simulink model "MaliLib"  (R2023b)
settings: Solver=FixedStepAuto  StartTime=0.0  StopTime=inf  RelTol=1e-3  EnableMultiTasking=on
settings Model: ExtModeTrigDuration=10  Creator=memoj  LastModifiedBy=memoj
settings OptimizationCC: EnhancedBackFolding=on  PassReuseOutputArgsAs=Individual arguments  ZeroExternalMemoryAtStartup=off  ZeroInternalMemoryAtStartup=off  MaxStackSize=64  OptimizeBlockOrder=speed  DifferentSizesBufferReuse=on  OptimizationCustomize=off  EfficientTunableParamExpr=on
settings DebuggingCC: ParameterTunabilityLossMsg=error
settings HardwareCC: ProdBitPerPointer=32  ProdBitPerSizeT=32  ProdBitPerPtrDiffT=32  ProdLargestAtomicInteger=Long  ProdLargestAtomicFloat=Double  ProdWordSize=32  ProdLongLongMode=on  ProdHWDeviceType=ARM Compatible->ARM Cortex
settings SFSimCC: MATLABDynamicMemAlloc=off
settings RTWCC: Description=Embedded Coder  SystemTargetFile=ert.tlc  HardwareBoard=STM32 Nucleo F767ZI  TemplateMakefile=ert_default_tmf  CustomSource=gpio_driver_mali.c  Toolchain=GNU Tools for ARM Embedded Processors
settings CodeAppCC: ForceParamTrailComments=on  IgnoreCustomStorageClasses=off  OperatorAnnotations=on  SimulinkDataObjDesc=on  SFDataObjDesc=on  InsertBlockDesc=on
settings ERTTargetCC: CodeReplacementLibrary=ARM Cortex-M  SupportNonInlinedSFcns=on  ExtModeTransport=3  ExtModeStaticAlloc=on  ExtModeStaticAllocSize=2000  ExtModeMexFile=ext_xcp  ExtModeIntrfLevel=Level2 - Open

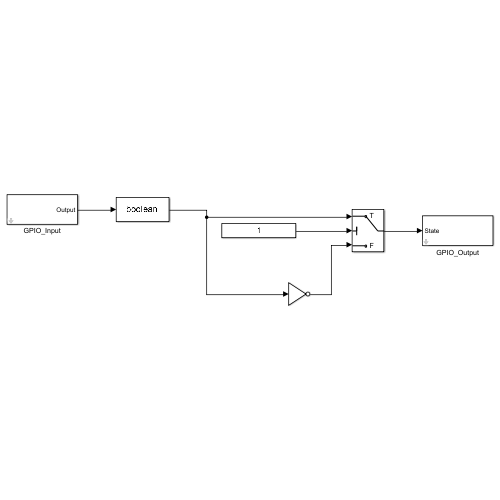
[thumbnail: Simulink's stored preview of the top-level diagram]
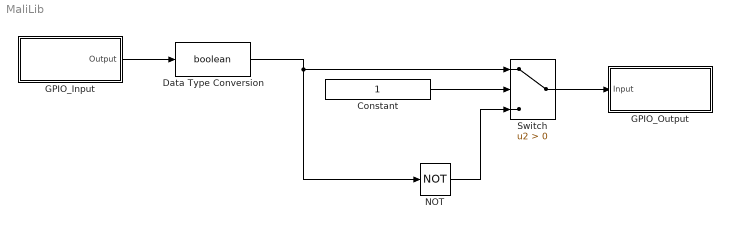
== system MaliLib ==
  Constant : Constant  OutDataTypeStr=boolean
  Data Type Conversion : DataTypeConversion  OutDataTypeStr=boolean  SaturateOnIntegerOverflow=off  RndMeth=Floor
  GPIO_Input : Subsystem  mask{port='C', pin=13, pull=PULLDOWN}
      mask prompts: pull "HS'mi LS'mi (PULLUP:HS ; PULLDOWN: LS)"
      mask TypeOptions pull: PULLUP | PULLDOWN | NOPULL
      mask Callback pull:
      | blk = gcb;  % maskelenmiş blokun kendisi
      |     val = get_param(blk, 'pull');
      | 
      |     % Alt blok ismi: PullConst
      |     switch val
      |         case 'PULLUP'
      |             set_param([blk '/PullConst'], 'Value', '1');
      |         case 'PULLDOWN'
      |             set_param([blk '/PullConst'], 'Value', '2');
      |         case 'NOPULL'
      |             set_param([blk '/PullConst'], 'Value', '0');
      |     end
  GPIO_Output : Subsystem  mask{port='B', pin=7, pull=Push-pull}
      mask prompts: pull "HS'mi LS'mi(Push-pull:HS ; Open-drain: LS)"
      mask TypeOptions pull: Push-pull | Open-drain
      mask Callback pull:
      | blk = gcb;  % maskelenmiş blokun kendisi
      |     val = get_param(blk, 'pull');
      | 
      |     % Alt blok ismi: PullConst
      |     switch val
      |         case 'Open-drain'
      |             set_param([blk '/PullConst'], 'Value', '1');
      |         case 'Push-pull'
      |             set_param([blk '/PullConst'], 'Value', '0');
      |     end
  NOT : Logic  Operator=NOT  IconShape=distinctive  AllPortsSameDT=off  OutDataTypeStr=boolean
  Switch : Switch  Criteria=u2 > Threshold  OutDataTypeStr=boolean  SaturateOnIntegerOverflow=off  InputSameDT=off
  wires:
  NOT/1 -> Switch/3
  Constant/1 -> Switch/2
  Data Type Conversion/1 -> NOT/1, Switch/1
  Switch/1 -> GPIO_Output/1(Input)
  GPIO_Input/1(Output) -> Data Type Conversion/1

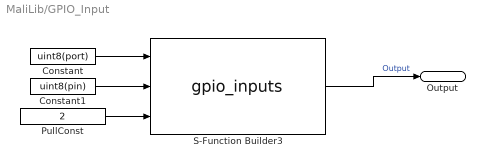
== system MaliLib/GPIO_Input ==
  Constant : Constant  Value=uint8(port)  OutDataTypeStr=uint8
  Constant1 : Constant  Value=uint8(pin)  OutDataTypeStr=uint8
  PullConst : Constant  Value=2  OutDataTypeStr=uint8
  S-Function Builder3 : S-Function  FunctionName=gpio_inputs  SFunctionModules=gpio_inputs_wrapper.c  SFunctionDeploymentMode=off  EnableBusSupport=off  mask(S-Function Builder){}
      mask help: Simulink:masks:SFunctionBuilder_MD
      mask init:
      | val = [[.9  0.75 0.75 1 1 .9 .9 1]',[1 1 0.75 0.75 .9 .9 1 .9]'];try , sys = get_param(gcb,'SfunBuilderFcnName');if isempty(sys), sys = get_param(gcb,'FunctionName'); end,catch, sys = get_param(gcb,'FunctionName'); end
      settings: CopyFcn=set_param(gcbh,'LinkStatus','none')  OpenFcn=sfunctionwizard(gcbh)
      mask Display:
      | plot(val(:,1),val(:,2))
      | disp(sys)
      | port_label('input',1,'port_ascii')
      | port_label('input',2,'pin')
      | port_label('input',3,'pull')
      | port_label('output',1,'readVal')
  Output : Outport  OutDataTypeStr=boolean
  wires:
  Constant/1 -> S-Function Builder3/1
  Constant1/1 -> S-Function Builder3/2
  S-Function Builder3/1 -> Output/1  "Output"
  PullConst/1 -> S-Function Builder3/3

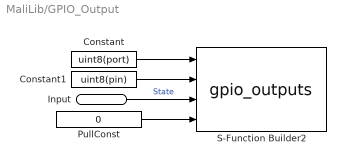
== system MaliLib/GPIO_Output ==
  Input : Inport  OutDataTypeStr=boolean
  Constant : Constant  Value=uint8(port)  OutDataTypeStr=uint8
  Constant1 : Constant  Value=uint8(pin)  OutDataTypeStr=uint8
  PullConst : Constant  Value=0  OutDataTypeStr=uint8
  S-Function Builder2 : S-Function  FunctionName=gpio_outputs  SFunctionModules=gpio_outputs_wrapper.c  SFunctionDeploymentMode=off  EnableBusSupport=off  mask(S-Function Builder){}
      mask help: Simulink:masks:SFunctionBuilder_MD
      mask init: same as MaliLib/GPIO_Input/S-Function Builder3
      settings: CopyFcn=set_param(gcbh,'LinkStatus','none')  OpenFcn=sfunctionwizard(gcbh)
      mask Display:
      | plot(val(:,1),val(:,2))
      | disp(sys)
      | port_label('input',1,'port_ascii')
      | port_label('input',2,'pin')
      | port_label('input',3,'state')
      | port_label('input',4,'pull')
  wires:
  Constant1/1 -> S-Function Builder2/2
  Constant/1 -> S-Function Builder2/1
  Input/1 -> S-Function Builder2/3  "State"
  PullConst/1 -> S-Function Builder2/4
